simulink model "combinedmodels"  (R2022b)
settings: Solver=VariableStepAuto  StartTime=0.0  StopTime=3600  RelTol=1e-3
libraries: sh_lib x46, spsThreePhaseVIMeasurementLib x36, spsThreePhaseSeriesRLCLoadLib x32, spsThreePhaseSeriesRLCBranchLib x32, fl_lib x27, nesl_utility x25, spsCurrentVoltageSimscapeInterfacegndLib x6, ee_lib x3, spsGroundLib x3, spsPower3phPhasorLib x3, SignalEditorBlockLib x3, spsThreePhaseParallelRLCBranchLib x3
(part 1 of 3)
settings Model: Creator=philip  LastModifiedBy=philip

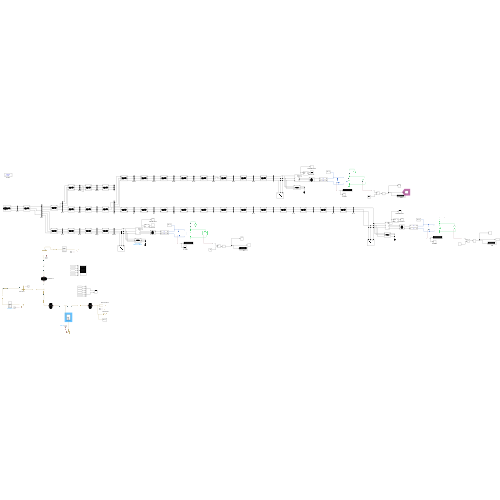
[thumbnail: Simulink's stored preview of the top-level diagram]
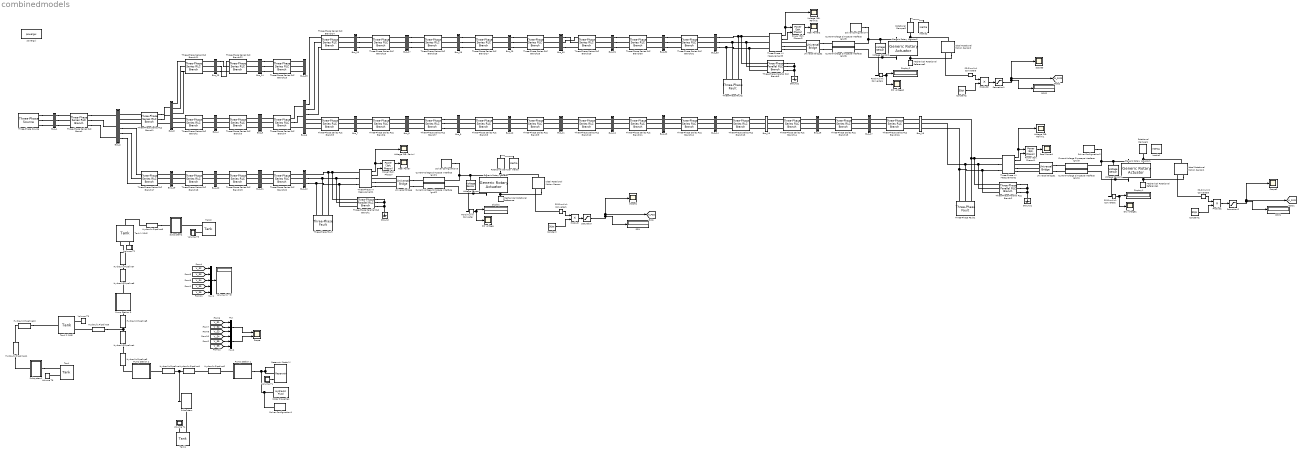
== system combinedmodels ==
  Bus_1 : Subsystem
  Bus_10 : Subsystem
  Bus_11 : Subsystem
  Bus_12 : Subsystem
  Bus_13 : Subsystem
  Bus_14 : Subsystem
  Bus_15 : Subsystem
  Bus_16 : Subsystem
  Bus_17 : Subsystem
  Bus_18 : Subsystem
  Bus_19 : Subsystem
  Bus_2 : Subsystem
  Bus_20 : Subsystem
  Bus_21 : Subsystem
  Bus_22 : Subsystem
  Bus_23 : Subsystem
  Bus_24 : Subsystem
  Bus_25 : Subsystem
  Bus_26 : Subsystem
  Bus_27 : Subsystem
  Bus_28 : Subsystem
  Bus_29 : Subsystem
  Bus_3 : Subsystem
  Bus_30 : Subsystem
  Bus_31 : Subsystem
  Bus_32 : Subsystem
  Bus_33 : Subsystem
  Bus_4 : Subsystem
  Bus_5 : Subsystem
  Bus_6 : Subsystem
  Bus_7 : Subsystem
  Bus_8 : Subsystem
  Bus_9 : Subsystem
  Constant : Constant  Value=30/pi  VectorParams1D=off
  Constant1 : Constant  Value=30/pi  VectorParams1D=off
  Constant2 : Constant  Value=30/pi  VectorParams1D=off
  Current-Voltage Simscape Interface (gnd){1..6} (6 alike) : spsCurrentVoltageSimscapeInterfacegndLib/Current-Voltage Simscape Interface (gnd)  DFT=off  Fmode=Low pass filter (continuous)  T=1e-6  Ts=50e-6  i0=0  v0=12660  Sd=Specialized Power Systems side  Measurements=off
      settings: LibrarySourceBlock=|
      | sps_lib/Utilities/Current-Voltage
      | Simscape Interface
      | (gnd)
  DC voltage : Scope
  DC voltage1 : Scope
  DC voltage2 : Scope
  Display : Display
  Display1 : Display
  Display2 : Display
  Generic Rotary Actuator : ee_lib/Electromechanical/Mechatronic Actuators/Generic Rotary Actuator  w_vec=[-1500, -1000, -500, 0, 500, 1000, 1500, 2000, 2500, 3000] rpm  T_vec=[3.8,3.5, 3, 2.5, 2, 1.5, 1, .5, 0, -.5,] N*m  Vrated=20000 V  eff=60  w_eff=2000 rpm  Pbase=1 W  pwm_or_av=1  J=0.1 kg*m^2  lam=1e-8 N*m/(rad/s)  i_specify=off  i_priority=None  i=0 A  i_nominal_specify=off  i_nominal_unit=A  i_nominal_value=1  t_specify=off  t_priority=None  t=0 N*m  t_nominal_specify=off  t_nominal_unit=N*m  t_nominal_value=1  w_specify=off  w_priority=Low  w=0 rpm  w_nominal_specify=off  w_nominal_unit=rpm  w_nominal_value=1  alpha=3.93e-3 1/K  Tmeas=25 degC  thermal_mass=100 J/K  Q_specify=off  Q_priority=None  Q=0 W  Q_nominal_specify=off  Q_nominal_unit=W  Q_nominal_value=1  temperature_specify=off  temperature_priority=High  temperature=300 K  temperature_nominal_specify=off  temperature_nominal_unit=K  temperature_nominal_value=1
      settings: InternalSimscapePortConfiguration="{\"Bottom\":[],\"Left\":[{\"id\":\"p\",\"label\":\"+\",\"type\":\"foundation.electrical.electrical\"},{\"id\":\"R\",\"label\":\"R\",\"type\":\"foundation.mechanical.rotational.rotational\"}],\"Right\":[{\"id\":\"n\",\"label\":\"-\",\"type\":\"foundation.electrical.electrical\"},{\"id\":\"C\",\"label\":\"C\",\"type\":\"foundation.mechanical.rotational.rotational\"}],\"Top\":[]}"
  Generic Rotary Actuator1 : ee_lib/Electromechanical/Mechatronic Actuators/Generic Rotary Actuator  w_vec=[-1500, -1000, -500, 0, 500, 1000, 1500, 2000, 2500, 3000] rpm  T_vec=[3.8,3.5, 3, 2.5, 2, 1.5, 1, .5, 0, -.5,] N*m  Vrated=20000 V  eff=60  w_eff=2000 rpm  Pbase=1 W  pwm_or_av=1  J=0.1 kg*m^2  lam=1e-8 N*m/(rad/s)  i_specify=off  i_priority=None  i=0 A  i_nominal_specify=off  i_nominal_unit=A  i_nominal_value=1  t_specify=off  t_priority=None  t=0 N*m  t_nominal_specify=off  t_nominal_unit=N*m  t_nominal_value=1  w_specify=off  w_priority=Low  w=0 rpm  w_nominal_specify=off  w_nominal_unit=rpm  w_nominal_value=1  alpha=3.93e-3 1/K  Tmeas=25 degC  thermal_mass=100 J/K  Q_specify=off  Q_priority=None  Q=0 W  Q_nominal_specify=off  Q_nominal_unit=W  Q_nominal_value=1  temperature_specify=off  temperature_priority=High  temperature=300 K  temperature_nominal_specify=off  temperature_nominal_unit=K  temperature_nominal_value=1
      settings: InternalSimscapePortConfiguration="{\"Bottom\":[],\"Left\":[{\"id\":\"p\",\"label\":\"+\",\"type\":\"foundation.electrical.electrical\"},{\"id\":\"R\",\"label\":\"R\",\"type\":\"foundation.mechanical.rotational.rotational\"}],\"Right\":[{\"id\":\"n\",\"label\":\"-\",\"type\":\"foundation.electrical.electrical\"},{\"id\":\"C\",\"label\":\"C\",\"type\":\"foundation.mechanical.rotational.rotational\"}],\"Top\":[]}"
  Generic Rotary Actuator2 : ee_lib/Electromechanical/Mechatronic Actuators/Generic Rotary Actuator  w_vec=[-1500, -1000, -500, 0, 500, 1000, 1500, 2000, 2500, 3000] rpm  T_vec=[3.8,3.5, 3, 2.5, 2, 1.5, 1, .5, 0, -.5,] N*m  Vrated=20000 V  eff=60  w_eff=2000 rpm  Pbase=1 W  pwm_or_av=1  J=0.1 kg*m^2  lam=1e-8 N*m/(rad/s)  i_specify=off  i_priority=None  i=0 A  i_nominal_specify=off  i_nominal_unit=A  i_nominal_value=1  t_specify=off  t_priority=None  t=0 N*m  t_nominal_specify=off  t_nominal_unit=N*m  t_nominal_value=1  w_specify=off  w_priority=Low  w=0 rpm  w_nominal_specify=off  w_nominal_unit=rpm  w_nominal_value=1  alpha=3.93e-3 1/K  Tmeas=25 degC  thermal_mass=100 J/K  Q_specify=off  Q_priority=None  Q=0 W  Q_nominal_specify=off  Q_nominal_unit=W  Q_nominal_value=1  temperature_specify=off  temperature_priority=High  temperature=300 K  temperature_nominal_specify=off  temperature_nominal_unit=K  temperature_nominal_value=1
      settings: InternalSimscapePortConfiguration="{\"Bottom\":[],\"Left\":[{\"id\":\"p\",\"label\":\"+\",\"type\":\"foundation.electrical.electrical\"},{\"id\":\"R\",\"label\":\"R\",\"type\":\"foundation.mechanical.rotational.rotational\"}],\"Right\":[{\"id\":\"n\",\"label\":\"-\",\"type\":\"foundation.electrical.electrical\"},{\"id\":\"C\",\"label\":\"C\",\"type\":\"foundation.mechanical.rotational.rotational\"}],\"Top\":[]}"
  Ground : spsGroundLib/Ground  LConnTagsString=a
  Ground1 : spsGroundLib/Ground  LConnTagsString=a
  Ground2 : spsGroundLib/Ground  LConnTagsString=a
  Hydraulic Pipeline : sh_lib/Pipelines/Hydraulic Pipeline  cs_type=foundation.enum.pipeCrossSection.circular  d_in=0.30 m  area=1e-4 m^2  D_h=1.12e-2 m  s_factor=64  length=18 m  length_ad=1 m  roughness=15e-6 m  Re_lam=2000  Re_turb=4000  wall_type=foundation.enum.chamber_spec.rigid  pr_r_coef=2e-12 m/Pa  time_const=0.01 s  k_sh=1.4  initial_pressure=0 Pa
      settings: InternalSimscapePortConfiguration="{\"Bottom\":[],\"Left\":[{\"id\":\"A\",\"label\":\"A\",\"type\":\"foundation.hydraulic.hydraulic\"}],\"Right\":[{\"id\":\"B\",\"label\":\"B\",\"type\":\"foundation.hydraulic.hydraulic\"}],\"Top\":[]}"
  Hydraulic Pipeline1 : sh_lib/Pipelines/Hydraulic Pipeline  cs_type=foundation.enum.pipeCrossSection.circular  d_in=0.15 m  area=1e-4 m^2  D_h=1.12e-2 m  s_factor=64  length=401 m  length_ad=1 m  roughness=15e-6 m  Re_lam=2000  Re_turb=4000  wall_type=foundation.enum.chamber_spec.rigid  pr_r_coef=2e-12 m/Pa  time_const=0.01 s  k_sh=1.4  initial_pressure=0 Pa
      settings: InternalSimscapePortConfiguration="{\"Bottom\":[],\"Left\":[{\"id\":\"A\",\"label\":\"A\",\"type\":\"foundation.hydraulic.hydraulic\"}],\"Right\":[{\"id\":\"B\",\"label\":\"B\",\"type\":\"foundation.hydraulic.hydraulic\"}],\"Top\":[]}"
  Hydraulic Pipeline10 : sh_lib/Pipelines/Hydraulic Pipeline  cs_type=foundation.enum.pipeCrossSection.circular  d_in=0.23 m  area=1e-4 m^2  D_h=1.12e-2 m  s_factor=64  length=6 m  length_ad=1 m  roughness=15e-6 m  Re_lam=2000  Re_turb=4000  wall_type=foundation.enum.chamber_spec.rigid  pr_r_coef=2e-12 m/Pa  time_const=0.01 s  k_sh=1.4  initial_pressure=0 Pa
      settings: InternalSimscapePortConfiguration="{\"Bottom\":[],\"Left\":[{\"id\":\"A\",\"label\":\"A\",\"type\":\"foundation.hydraulic.hydraulic\"}],\"Right\":[{\"id\":\"B\",\"label\":\"B\",\"type\":\"foundation.hydraulic.hydraulic\"}],\"Top\":[]}"
  Hydraulic Pipeline11 : sh_lib/Pipelines/Hydraulic Pipeline  cs_type=foundation.enum.pipeCrossSection.circular  d_in=0.30 m  area=1e-4 m^2  D_h=1.12e-2 m  s_factor=64  length=13 m  length_ad=1 m  roughness=15e-6 m  Re_lam=2000  Re_turb=4000  wall_type=foundation.enum.chamber_spec.rigid  pr_r_coef=2e-12 m/Pa  time_const=0.01 s  k_sh=1.4  initial_pressure=0 Pa
      settings: InternalSimscapePortConfiguration="{\"Bottom\":[],\"Left\":[{\"id\":\"A\",\"label\":\"A\",\"type\":\"foundation.hydraulic.hydraulic\"}],\"Right\":[{\"id\":\"B\",\"label\":\"B\",\"type\":\"foundation.hydraulic.hydraulic\"}],\"Top\":[]}"
  Hydraulic Pipeline2 : sh_lib/Pipelines/Hydraulic Pipeline  cs_type=foundation.enum.pipeCrossSection.circular  d_in=0.15 m  area=1e-4 m^2  D_h=1.12e-2 m  s_factor=64  length=15 m  length_ad=1 m  roughness=15e-6 m  Re_lam=2000  Re_turb=4000  wall_type=foundation.enum.chamber_spec.rigid  pr_r_coef=2e-12 m/Pa  time_const=0.01 s  k_sh=1.4  initial_pressure=0 Pa
      settings: InternalSimscapePortConfiguration="{\"Bottom\":[],\"Left\":[{\"id\":\"A\",\"label\":\"A\",\"type\":\"foundation.hydraulic.hydraulic\"}],\"Right\":[{\"id\":\"B\",\"label\":\"B\",\"type\":\"foundation.hydraulic.hydraulic\"}],\"Top\":[]}"
  Hydraulic Pipeline3 : sh_lib/Pipelines/Hydraulic Pipeline  cs_type=foundation.enum.pipeCrossSection.circular  d_in=0.25 m  area=1e-4 m^2  D_h=1.12e-2 m  s_factor=64  length=1087 m  length_ad=1 m  roughness=15e-6 m  Re_lam=2000  Re_turb=4000  wall_type=foundation.enum.chamber_spec.rigid  pr_r_coef=2e-12 m/Pa  time_const=0.01 s  k_sh=1.4  initial_pressure=0 Pa
      settings: InternalSimscapePortConfiguration="{\"Bottom\":[],\"Left\":[{\"id\":\"A\",\"label\":\"A\",\"type\":\"foundation.hydraulic.hydraulic\"}],\"Right\":[{\"id\":\"B\",\"label\":\"B\",\"type\":\"foundation.hydraulic.hydraulic\"}],\"Top\":[]}"
  Hydraulic Pipeline4 : sh_lib/Pipelines/Hydraulic Pipeline  cs_type=foundation.enum.pipeCrossSection.circular  d_in=0.15 m  area=1e-4 m^2  D_h=1.12e-2 m  s_factor=64  length=1002 m  length_ad=1 m  roughness=15e-6 m  Re_lam=2000  Re_turb=4000  wall_type=foundation.enum.chamber_spec.rigid  pr_r_coef=2e-12 m/Pa  time_const=0.01 s  k_sh=1.4  initial_pressure=0 Pa
      settings: InternalSimscapePortConfiguration="{\"Bottom\":[],\"Left\":[{\"id\":\"A\",\"label\":\"A\",\"type\":\"foundation.hydraulic.hydraulic\"}],\"Right\":[{\"id\":\"B\",\"label\":\"B\",\"type\":\"foundation.hydraulic.hydraulic\"}],\"Top\":[]}"
  Hydraulic Pipeline5 : sh_lib/Pipelines/Hydraulic Pipeline  cs_type=foundation.enum.pipeCrossSection.circular  d_in=0.10 m  area=1e-4 m^2  D_h=1.12e-2 m  s_factor=64  length=846 m  length_ad=1 m  roughness=15e-6 m  Re_lam=2000  Re_turb=4000  wall_type=foundation.enum.chamber_spec.rigid  pr_r_coef=2e-12 m/Pa  time_const=0.01 s  k_sh=1.4  initial_pressure=0 Pa
      settings: InternalSimscapePortConfiguration="{\"Bottom\":[],\"Left\":[{\"id\":\"A\",\"label\":\"A\",\"type\":\"foundation.hydraulic.hydraulic\"}],\"Right\":[{\"id\":\"B\",\"label\":\"B\",\"type\":\"foundation.hydraulic.hydraulic\"}],\"Top\":[]}"
  Hydraulic Pipeline6 : sh_lib/Pipelines/Hydraulic Pipeline  cs_type=foundation.enum.pipeCrossSection.circular  d_in=0.25 m  area=1e-4 m^2  D_h=1.12e-2 m  s_factor=64  length=44 m  length_ad=1 m  roughness=15e-6 m  Re_lam=2000  Re_turb=4000  wall_type=foundation.enum.chamber_spec.rigid  pr_r_coef=2e-12 m/Pa  time_const=0.01 s  k_sh=1.4  initial_pressure=0 Pa
      settings: InternalSimscapePortConfiguration="{\"Bottom\":[],\"Left\":[{\"id\":\"A\",\"label\":\"A\",\"type\":\"foundation.hydraulic.hydraulic\"}],\"Right\":[{\"id\":\"B\",\"label\":\"B\",\"type\":\"foundation.hydraulic.hydraulic\"}],\"Top\":[]}"
  Hydraulic Pipeline7 : sh_lib/Pipelines/Hydraulic Pipeline  cs_type=foundation.enum.pipeCrossSection.circular  d_in=0.25 m  area=1e-4 m^2  D_h=1.12e-2 m  s_factor=64  length=18 m  length_ad=1 m  roughness=15e-6 m  Re_lam=2000  Re_turb=4000  wall_type=foundation.enum.chamber_spec.rigid  pr_r_coef=2e-12 m/Pa  time_const=0.01 s  k_sh=1.4  initial_pressure=0 Pa
      settings: InternalSimscapePortConfiguration="{\"Bottom\":[],\"Left\":[{\"id\":\"A\",\"label\":\"A\",\"type\":\"foundation.hydraulic.hydraulic\"}],\"Right\":[{\"id\":\"B\",\"label\":\"B\",\"type\":\"foundation.hydraulic.hydraulic\"}],\"Top\":[]}"
  Hydraulic Pipeline8 : sh_lib/Pipelines/Hydraulic Pipeline  cs_type=foundation.enum.pipeCrossSection.circular  d_in=0.10 m  area=1e-4 m^2  D_h=1.12e-2 m  s_factor=64  length=16 m  length_ad=1 m  roughness=15e-6 m  Re_lam=2000  Re_turb=4000  wall_type=foundation.enum.chamber_spec.rigid  pr_r_coef=2e-12 m/Pa  time_const=0.01 s  k_sh=1.4  initial_pressure=0 Pa
      settings: InternalSimscapePortConfiguration="{\"Bottom\":[],\"Left\":[{\"id\":\"A\",\"label\":\"A\",\"type\":\"foundation.hydraulic.hydraulic\"}],\"Right\":[{\"id\":\"B\",\"label\":\"B\",\"type\":\"foundation.hydraulic.hydraulic\"}],\"Top\":[]}"
  Hydraulic Pipeline9 : sh_lib/Pipelines/Hydraulic Pipeline  cs_type=foundation.enum.pipeCrossSection.circular  d_in=0.20 m  area=1e-4 m^2  D_h=1.12e-2 m  s_factor=64  length=1003 m  length_ad=1 m  roughness=15e-6 m  Re_lam=2000  Re_turb=4000  wall_type=foundation.enum.chamber_spec.rigid  pr_r_coef=2e-12 m/Pa  time_const=0.01 s  k_sh=1.4  initial_pressure=0 Pa
      settings: InternalSimscapePortConfiguration="{\"Bottom\":[],\"Left\":[{\"id\":\"A\",\"label\":\"A\",\"type\":\"foundation.hydraulic.hydraulic\"}],\"Right\":[{\"id\":\"B\",\"label\":\"B\",\"type\":\"foundation.hydraulic.hydraulic\"}],\"Top\":[]}"
  Ideal Rotational Motion Sensor : fl_lib/Mechanical/Mechanical Sensors/Ideal Rotational Motion Sensor  reference=foundation.enum.MeasurementReference.difference  acceleration_port=false  velocity_port=true  position_port=false  wrap_angle=false  offset=0 rad
      settings: InternalSimscapePortConfiguration="{\"Bottom\":[],\"Left\":[{\"id\":\"R\",\"label\":\"R\",\"type\":\"foundation.mechanical.rotational.rotational\"}],\"Right\":[{\"id\":\"C\",\"label\":\"C\",\"type\":\"foundation.mechanical.rotational.rotational\"},{\"id\":\"W\",\"label\":\"W\",\"type\":\"output\"}],\"Top\":[]}"
  Ideal Rotational Motion Sensor1 : fl_lib/Mechanical/Mechanical Sensors/Ideal Rotational Motion Sensor  reference=foundation.enum.MeasurementReference.difference  acceleration_port=false  velocity_port=true  position_port=false  wrap_angle=false  offset=0 rad
      settings: InternalSimscapePortConfiguration="{\"Bottom\":[],\"Left\":[{\"id\":\"R\",\"label\":\"R\",\"type\":\"foundation.mechanical.rotational.rotational\"}],\"Right\":[{\"id\":\"C\",\"label\":\"C\",\"type\":\"foundation.mechanical.rotational.rotational\"},{\"id\":\"W\",\"label\":\"W\",\"type\":\"output\"}],\"Top\":[]}"
  Ideal Rotational Motion Sensor2 : fl_lib/Mechanical/Mechanical Sensors/Ideal Rotational Motion Sensor  reference=foundation.enum.MeasurementReference.difference  acceleration_port=false  velocity_port=true  position_port=false  wrap_angle=false  offset=0 rad
      settings: InternalSimscapePortConfiguration="{\"Bottom\":[],\"Left\":[{\"id\":\"R\",\"label\":\"R\",\"type\":\"foundation.mechanical.rotational.rotational\"}],\"Right\":[{\"id\":\"C\",\"label\":\"C\",\"type\":\"foundation.mechanical.rotational.rotational\"},{\"id\":\"W\",\"label\":\"W\",\"type\":\"output\"}],\"Top\":[]}"
  Inertia : fl_lib/Mechanical/Rotational Elements/Inertia  inertia=0.1 kg*m^2  num_ports=foundation.enum.numPorts2.one  w_specify=off  w_priority=High  w=0 rad/s  w_nominal_specify=off  w_nominal_unit=rad/s  w_nominal_value=1  t_specify=off  t_priority=None  t=0 N*m  t_nominal_specify=off  t_nominal_unit=N*m  t_nominal_value=1
  Inertia1 : fl_lib/Mechanical/Rotational Elements/Inertia  inertia=0.1 kg*m^2  num_ports=foundation.enum.numPorts2.one  w_specify=off  w_priority=High  w=0 rad/s  w_nominal_specify=off  w_nominal_unit=rad/s  w_nominal_value=1  t_specify=off  t_priority=None  t=0 N*m  t_nominal_specify=off  t_nominal_unit=N*m  t_nominal_value=1
  Inertia2 : fl_lib/Mechanical/Rotational Elements/Inertia  inertia=0.1 kg*m^2  num_ports=foundation.enum.numPorts2.one  w_specify=off  w_priority=High  w=0 rad/s  w_nominal_specify=off  w_nominal_unit=rad/s  w_nominal_value=1  t_specify=off  t_priority=None  t=0 N*m  t_nominal_specify=off  t_nominal_unit=N*m  t_nominal_value=1
  Mechanical Rotational Reference : fl_lib/Mechanical/Rotational Elements/Mechanical Rotational Reference
  Mechanical Rotational Reference1 : fl_lib/Mechanical/Rotational Elements/Mechanical Rotational Reference
  Mechanical Rotational Reference2 : fl_lib/Mechanical/Rotational Elements/Mechanical Rotational Reference
  Mux : Mux  Inputs=3
  Mux1 : Mux  Inputs=5
  Mux2 : Mux  Inputs=3
  PS-Simulink Converter : nesl_utility/PS-Simulink Converter  PhysicalDomain=network_engine_domain  SubClassName=ps_output  LeftPortType=input  RightPortType=output  PseudoPeriodic=off  Frequencies=[]  VectorFormat=1-D array  Unit=inherit  AffineConversion=off
  PS-Simulink Converter1 : nesl_utility/PS-Simulink Converter  PhysicalDomain=network_engine_domain  SubClassName=ps_output  LeftPortType=input  RightPortType=output  PseudoPeriodic=off  Frequencies=[]  VectorFormat=inherit  Unit=inherit  AffineConversion=off
  PS-Simulink Converter2 : nesl_utility/PS-Simulink Converter  PhysicalDomain=network_engine_domain  SubClassName=ps_output  LeftPortType=input  RightPortType=output  PseudoPeriodic=off  Frequencies=[]  VectorFormat=1-D array  Unit=inherit  AffineConversion=off
  PS-Simulink Converter3 : nesl_utility/PS-Simulink Converter  PhysicalDomain=network_engine_domain  SubClassName=ps_output  LeftPortType=input  RightPortType=output  PseudoPeriodic=off  Frequencies=[]  VectorFormat=inherit  Unit=inherit  AffineConversion=off
  PS-Simulink Converter4 : nesl_utility/PS-Simulink Converter  PhysicalDomain=network_engine_domain  SubClassName=ps_output  LeftPortType=input  RightPortType=output  PseudoPeriodic=off  Frequencies=[]  VectorFormat=1-D array  Unit=inherit  AffineConversion=off
  PS-Simulink Converter5 : nesl_utility/PS-Simulink Converter  PhysicalDomain=network_engine_domain  SubClassName=ps_output  LeftPortType=input  RightPortType=output  PseudoPeriodic=off  Frequencies=[]  VectorFormat=inherit  Unit=inherit  AffineConversion=off
  "Power (3ph, Phasor)" : spsPower3phPhasorLib/Power (3ph, Phasor)
      settings: LibrarySourceBlock=|
      | sps_lib/Sensors and Measurements/Power
      | (3ph, Phasor)
  "Power (3ph, Phasor)1" : spsPower3phPhasorLib/Power (3ph, Phasor)
      settings: LibrarySourceBlock=|
      | sps_lib/Sensors and Measurements/Power
      | (3ph, Phasor)
  "Power (3ph, Phasor)2" : spsPower3phPhasorLib/Power (3ph, Phasor)
      settings: LibrarySourceBlock=|
      | sps_lib/Sensors and Measurements/Power
      | (3ph, Phasor)
  Product : Product
  Product1 : Product
  Product2 : Product
  Pump Station 1 : Subsystem  Tag=PublishSubsystem
      mask Display:
      | plot(sin(0:0.5:4.5*pi)*0.9, cos(0:0.5:4.5*pi)*0.9+1.5)
      | plot(sin(0:0.5:4.5*pi)*0.5, cos(0:0.5:4.5*pi)*0.5+1.5)
      | plot(sin(0:0.5:4.5*pi)*0.9, cos(0:0.5:4.5*pi)*0.9-1.5)
      | plot(sin(0:0.5:4.5*pi)*0.5, cos(0:0.5:4.5*pi)*0.5-1.5)
      | 
      | plot([0 -0.9],[1.5 1.5-0.9])
      | plot([0 -0.9],[1.5 1.5-0.9]*-1)
      | 
      | plot([0.45 0.45 0.325 0.325]*2,[1.5 1.5-1.0 1.5-1.0 1.5-0.55])
      | plot([0.45 0.45 0.325 0.325]*2,[1.5 1.5-0.9 1.5-0.9 1.5-0.55]*-1)
      | 
      | plot([2.2 0.95]*-1,[0 0])
      | plot([2.2 0.95],[0 0])
      | 
      | plot([0.95 0.95]*-1,[-0.6 0.6])
      | plot([0.8 0.8],[-0.55 0.55])
      | 
      | 
      | color('white');plot(-3,-2.5);plot(3,2.5);
      | color('red');
      | port_label('LConn',1,'T');
      | port_label('RConn',1,'P');
  Pump Station 2 : Subsystem  Tag=PublishSubsystem
      mask Display:
      | plot(sin(0:0.5:4.5*pi)*0.9, cos(0:0.5:4.5*pi)*0.9+1.5)
      | plot(sin(0:0.5:4.5*pi)*0.5, cos(0:0.5:4.5*pi)*0.5+1.5)
      | plot(sin(0:0.5:4.5*pi)*0.9, cos(0:0.5:4.5*pi)*0.9-1.5)
      | plot(sin(0:0.5:4.5*pi)*0.5, cos(0:0.5:4.5*pi)*0.5-1.5)
      | 
      | plot([0 -0.9],[1.5 1.5-0.9])
      | plot([0 -0.9],[1.5 1.5-0.9]*-1)
      | 
      | plot([0.45 0.45 0.325 0.325]*2,[1.5 1.5-1.0 1.5-1.0 1.5-0.55])
      | plot([0.45 0.45 0.325 0.325]*2,[1.5 1.5-0.9 1.5-0.9 1.5-0.55]*-1)
      | 
      | plot([2.2 0.95]*-1,[0 0])
      | plot([2.2 0.95],[0 0])
      | 
      | plot([0.95 0.95]*-1,[-0.6 0.6])
      | plot([0.8 0.8],[-0.55 0.55])
      | 
      | 
      | color('white');plot(-3,-2.5);plot(3,2.5);
      | color('red');
      | port_label('LConn',1,'T');
      | port_label('RConn',1,'P');
  Pump Station 3 : Subsystem  Tag=PublishSubsystem
      mask Display:
      | plot(sin(0:0.5:4.5*pi)*0.9, cos(0:0.5:4.5*pi)*0.9+1.5)
      | plot(sin(0:0.5:4.5*pi)*0.5, cos(0:0.5:4.5*pi)*0.5+1.5)
      | plot(sin(0:0.5:4.5*pi)*0.9, cos(0:0.5:4.5*pi)*0.9-1.5)
      | plot(sin(0:0.5:4.5*pi)*0.5, cos(0:0.5:4.5*pi)*0.5-1.5)
      | 
      | plot([0 -0.9],[1.5 1.5-0.9])
      | plot([0 -0.9],[1.5 1.5-0.9]*-1)
      | 
      | plot([0.45 0.45 0.325 0.325]*2,[1.5 1.5-1.0 1.5-1.0 1.5-0.55])
      | plot([0.45 0.45 0.325 0.325]*2,[1.5 1.5-0.9 1.5-0.9 1.5-0.55]*-1)
      | 
      | plot([2.2 0.95]*-1,[0 0])
      | plot([2.2 0.95],[0 0])
      | 
      | plot([0.95 0.95]*-1,[-0.6 0.6])
      | plot([0.8 0.8],[-0.55 0.55])
      | 
      | 
      | color('white');plot(-3,-2.5);plot(3,2.5);
      | color('red');
      | port_label('LConn',1,'T');
      | port_label('RConn',1,'P');
  RPM : Display
  RPM1 : Display
  RPM2 : Display
  Real Power : Scope
  Real Power1 : Scope
  Real Power2 : Scope
  Reservoir (Node 1) : sh_lib/Hydraulic Utilities/Reservoir  press=0 Pa  init_volume=200 m^3  ret_diam=0.15 m  loss_coeff=1
      settings: InternalSimscapePortConfiguration="{\"Bottom\":[],\"Left\":[{\"id\":\"V\",\"label\":\"V\",\"type\":\"output\"},{\"id\":\"P\",\"label\":\"P\",\"type\":\"foundation.hydraulic.hydraulic\"},{\"id\":\"R\",\"label\":\"R\",\"type\":\"foundation.hydraulic.hydraulic\"}],\"Right\":[],\"Top\":[]}"
  Rotational Damper : fl_lib/Mechanical/Rotational Elements/Rotational Damper  D=0.001 N*m/(rad/s)  w_specify=off  w_priority=None  w=0 rad/s  w_nominal_specify=off  w_nominal_unit=rad/s  w_nominal_value=1  t_specify=off  t_priority=None  t=0 N*m  t_nominal_specify=off  t_nominal_unit=N*m  t_nominal_value=1
  Rotational Damper1 : fl_lib/Mechanical/Rotational Elements/Rotational Damper  D=0.001 N*m/(rad/s)  w_specify=off  w_priority=None  w=0 rad/s  w_nominal_specify=off  w_nominal_unit=rad/s  w_nominal_value=1  t_specify=off  t_priority=None  t=0 N*m  t_nominal_specify=off  t_nominal_unit=N*m  t_nominal_value=1
  Rotational Damper2 : fl_lib/Mechanical/Rotational Elements/Rotational Damper  D=0.001 N*m/(rad/s)  w_specify=off  w_priority=None  w=0 rad/s  w_nominal_specify=off  w_nominal_unit=rad/s  w_nominal_value=1  t_specify=off  t_priority=None  t=0 N*m  t_nominal_specify=off  t_nominal_unit=N*m  t_nominal_value=1
  Saturation : Saturate  UpperLimit=2500  LowerLimit=0  OutMin=[0]  OutMax=[2500]
  Saturation1 : Saturate  UpperLimit=2500  LowerLimit=0  OutMin=[0]  OutMax=[2500]
  Saturation2 : Saturate  UpperLimit=2500  LowerLimit=0  OutMin=[0]  OutMax=[2500]
  Scope : Scope  NumInputPorts=2
  Scope1 : Scope
  Scope2 : Scope
  Scope3 : Scope
  Solver Configuration1 : nesl_utility/Solver Configuration  PhysicalDomain=network_engine_domain  SubClassName=solver  LeftPortType=input  RightPortType=generic  Tones=[]  Harmonics=[]  SimulateNoise=off  Profile=off  UseLocalSampling=off  EnableSwitchedLinearOptims=on  FrequencyDomain=off  UseCCode=off  RelTol=0.001  AbsTol=1e-06  MinStep=1e-09  ToWorkspace=off  RevertToSquareIcSolve=off  NumHomotopyIterations=100  PhasorMode=off  PhasorModeNumHarmonics=1  ConsistencySolver=NEWTON_XTOL_AFTER_FTOL  IndexReductionMethod=DerivativeReplacement  DoDC=off  ResidualTolerance=1e-9  ConsistencyTolSource=GLOBAL  ConsistencyAbsTol=0.001  ConsistencyRelTol=0.001  ConsistencyTolFactor=0.034  UseLocalSolver=off  LocalSolverChoice=NE_BACKWARD_EULER_ADVANCER  ResolveIndetEquations=on  FunctionEvalNumThread=1  LocalSolverSampleTime=.001  DoFixedCost=on  MaxNonlinIter=3  MaxModeIter=2  ComputeImpulses=off  ImpulseIterations=2  LinearAlgebra=auto  LinearAlgebraNumThread=0  EquationFormulation=NE_TIME_EF  DelaysMemoryBudget=1024  AutomaticFiltering=off  FilteringTimeConstant=0.0001  PartitionStorageMethod=AS_NEEDED  PartitionMemoryBudget=1024  PartitionMethod=FAST
  Solver Configuration2 : nesl_utility/Solver Configuration  PhysicalDomain=network_engine_domain  SubClassName=solver  LeftPortType=input  RightPortType=generic  Tones=[]  Harmonics=[]  SimulateNoise=off  Profile=off  UseLocalSampling=off  EnableSwitchedLinearOptims=on  FrequencyDomain=off  UseCCode=off  RelTol=0.001  AbsTol=1e-06  MinStep=1e-09  ToWorkspace=off  RevertToSquareIcSolve=off  NumHomotopyIterations=100  PhasorMode=off  PhasorModeNumHarmonics=1  ConsistencySolver=NEWTON_FTOL  IndexReductionMethod=DerivativeReplacement  DoDC=off  ResidualTolerance=1e-09  ConsistencyTolSource=GLOBAL  ConsistencyAbsTol=0.001  ConsistencyRelTol=0.001  ConsistencyTolFactor=0.001  UseLocalSolver=off  LocalSolverChoice=NE_BACKWARD_EULER_ADVANCER  ResolveIndetEquations=on  FunctionEvalNumThread=1  LocalSolverSampleTime=0.001  DoFixedCost=off  MaxNonlinIter=3  MaxModeIter=2  ComputeImpulses=off  ImpulseIterations=2  LinearAlgebra=auto  LinearAlgebraNumThread=0  EquationFormulation=NE_TIME_EF  DelaysMemoryBudget=1024  AutomaticFiltering=on  FilteringTimeConstant=0.001  PartitionStorageMethod=AS_NEEDED  PartitionMemoryBudget=1024  PartitionMethod=ROBUST
  Solver Configuration3 : nesl_utility/Solver Configuration  PhysicalDomain=network_engine_domain  SubClassName=solver  LeftPortType=input  RightPortType=generic  Tones=[]  Harmonics=[]  SimulateNoise=off  Profile=off  UseLocalSampling=off  EnableSwitchedLinearOptims=on  FrequencyDomain=off  UseCCode=off  RelTol=0.001  AbsTol=1e-06  MinStep=1e-09  ToWorkspace=off  RevertToSquareIcSolve=off  NumHomotopyIterations=100  PhasorMode=off  PhasorModeNumHarmonics=1  ConsistencySolver=NEWTON_FTOL  IndexReductionMethod=DerivativeReplacement  DoDC=off  ResidualTolerance=1e-09  ConsistencyTolSource=GLOBAL  ConsistencyAbsTol=0.001  ConsistencyRelTol=0.001  ConsistencyTolFactor=0.001  UseLocalSolver=off  LocalSolverChoice=NE_BACKWARD_EULER_ADVANCER  ResolveIndetEquations=on  FunctionEvalNumThread=1  LocalSolverSampleTime=0.001  DoFixedCost=off  MaxNonlinIter=3  MaxModeIter=2  ComputeImpulses=off  ImpulseIterations=2  LinearAlgebra=auto  LinearAlgebraNumThread=0  EquationFormulation=NE_TIME_EF  DelaysMemoryBudget=1024  AutomaticFiltering=on  FilteringTimeConstant=0.001  PartitionStorageMethod=AS_NEEDED  PartitionMemoryBudget=1024  PartitionMethod=ROBUST
  Solver Configuration4 : nesl_utility/Solver Configuration  PhysicalDomain=network_engine_domain  SubClassName=solver  LeftPortType=input  RightPortType=generic  Tones=[]  Harmonics=[]  SimulateNoise=off  Profile=off  UseLocalSampling=off  EnableSwitchedLinearOptims=on  FrequencyDomain=off  UseCCode=off  RelTol=0.001  AbsTol=1e-06  MinStep=1e-09  ToWorkspace=off  RevertToSquareIcSolve=off  NumHomotopyIterations=100  PhasorMode=off  PhasorModeNumHarmonics=1  ConsistencySolver=NEWTON_FTOL  IndexReductionMethod=DerivativeReplacement  DoDC=off  ResidualTolerance=1e-09  ConsistencyTolSource=GLOBAL  ConsistencyAbsTol=0.001  ConsistencyRelTol=0.001  ConsistencyTolFactor=0.001  UseLocalSolver=off  LocalSolverChoice=NE_BACKWARD_EULER_ADVANCER  ResolveIndetEquations=on  FunctionEvalNumThread=1  LocalSolverSampleTime=0.001  DoFixedCost=off  MaxNonlinIter=3  MaxModeIter=2  ComputeImpulses=off  ImpulseIterations=2  LinearAlgebra=auto  LinearAlgebraNumThread=0  EquationFormulation=NE_TIME_EF  DelaysMemoryBudget=1024  AutomaticFiltering=on  FilteringTimeConstant=0.001  PartitionStorageMethod=AS_NEEDED  PartitionMemoryBudget=1024  PartitionMethod=ROBUST
  Subsystem : Subsystem
      settings: PortSchema="{\"entries\":[{\"content\":{\"sides\":[{\"content\":{\"connectorIds\":[\"LConn1\"]},\"type\":\"ConnectorPlacement.EquallySpacedRectSide\",\"uuid\":\"c5da6f35-8fa4-48b7-8a4a-4ae9db04ca9d\"},{\"content\":{\"connectorIds\":[],\"side\":\"RIGHT\"},\"type\":\"ConnectorPlacement.EquallySpacedRectSide\",\"uuid\":\"484dc1ab-2dc7-464f-80da-36af203a6e69\"},{\"content\":{\"connectorIds\":[],\"side\":\"TOP\"},\"type\":\"ConnectorPlacement.EquallySpacedRectSide\",\"uuid\":\"15bf6548-86e0-4373-a220-3fe0e1067d73\"},{\"content\":{\"connectorIds\":[\"RConn1\"],\"side\":\"BOTTOM\"},\"type\":\"ConnectorPlacement.EquallySpacedRectSide\",\"uuid\":\"b94051b1-e6bf-4793-98e6-5d6956093d36\"}]},\"type\":\"ConnectorPlacement.EquallySpacedConnector\",\"uuid\":\"b1159124-f196-4e4e-b402-5d78480e647c\"}],\"packageUris\":[\"http://schema.mathworks.com/mf0/Connector/R2020b\"],\"version\":\"1.0\"}"
  Subsystem1 : Subsystem
  Subsystem2 : Subsystem
  Tank : sh_lib/Low-Pressure Blocks/Tank  press=0 Pa  level_spec=1  tank_area=0.8 m^2  fluid_volume_tab=[0, .0028, .0065, .0114, .0176, .0252, .0344, .0436, .0512, .0574, .0623, .066, .0688, .0707, .072, .0727] m^3  fluid_level_tab=[0, .02, .04, .06, .08, .1, .12, .14, .16, .18, .2, .22, .24, .26, .28, .3] m  interp_method=1  extrap_method=1  pipe_diam=0.10 m  loss_coeff=1.2  g=9.80665 m/s^2  min_level=1e-3 m  fluid_level_check=0  volume_specify=off  volume_priority=High  volume=20 l  volume_nominal_specify=off  volume_nominal_unit=l  volume_nominal_value=1  level_specify=off  level_priority=None  level=0.025 m  level_nominal_specify=off  level_nominal_unit=m  level_nominal_value=1  pipe_diam_A=0.02 m  loss_coeff_A=1.2  height_B=0.8 m  pipe_diam_B=0.02 m  loss_coeff_B=1.2  height_C=0.8 m  pipe_diam_C=0.02 m  loss_coeff_C=1.2
      settings: InternalSimscapePortConfiguration="{\"Bottom\":[],\"Left\":[],\"Right\":[{\"id\":\"V\",\"label\":\"V\",\"type\":\"output\"},{\"id\":\"T\",\"label\":\"T\",\"type\":\"foundation.hydraulic.hydraulic\"}],\"Top\":[]}"
  Tank 1 (N10) : sh_lib/Low-Pressure Blocks/Tank  press=0 Pa  level_spec=1  tank_area=0.8 m^2  fluid_volume_tab=[0, .0028, .0065, .0114, .0176, .0252, .0344, .0436, .0512, .0574, .0623, .066, .0688, .0707, .072, .0727] m^3  fluid_level_tab=[0, .02, .04, .06, .08, .1, .12, .14, .16, .18, .2, .22, .24, .26, .28, .3] m  interp_method=1  extrap_method=1  pipe_diam=0.02 m  loss_coeff=1.2  g=9.80665 m/s^2  min_level=1e-3 m  fluid_level_check=0  volume_specify=off  volume_priority=High  volume=100 m^3  volume_nominal_specify=off  volume_nominal_unit=l  volume_nominal_value=1  level_specify=off  level_priority=None  level=station_3.fluid_level m  level_nominal_specify=off  level_nominal_unit=m  level_nominal_value=1  pipe_diam_A=0.25 m  loss_coeff_A=1.2  height_B=0.8 m  pipe_diam_B=0.10 m  loss_coeff_B=1.2  height_C=0.8 m  pipe_diam_C=0.02 m  loss_coeff_C=1.2
      settings: InternalSimscapePortConfiguration="{\"Bottom\":[],\"Left\":[{\"id\":\"B\",\"label\":\"B\",\"type\":\"foundation.hydraulic.hydraulic\"}],\"Right\":[{\"id\":\"V\",\"label\":\"V\",\"type\":\"output\"},{\"id\":\"A\",\"label\":\"A\",\"type\":\"foundation.hydraulic.hydraulic\"}],\"Top\":[]}"
  Tank 2 (N13) : sh_lib/Low-Pressure Blocks/Tank  press=0 Pa  level_spec=1  tank_area=0.8 m^2  fluid_volume_tab=[0, .0028, .0065, .0114, .0176, .0252, .0344, .0436, .0512, .0574, .0623, .066, .0688, .0707, .072, .0727] m^3  fluid_level_tab=[0, .02, .04, .06, .08, .1, .12, .14, .16, .18, .2, .22, .24, .26, .28, .3] m  interp_method=1  extrap_method=1  pipe_diam=0.02 m  loss_coeff=1.2  g=9.80665 m/s^2  min_level=1e-3 m  fluid_level_check=0  volume_specify=off  volume_priority=High  volume=100 m^3  volume_nominal_specify=off  volume_nominal_unit=l  volume_nominal_value=1  level_specify=off  level_priority=None  level=station_2.fluid_level m  level_nominal_specify=off  level_nominal_unit=m  level_nominal_value=1  pipe_diam_A=0.20 m  loss_coeff_A=1.2  height_B=0.8 m  pipe_diam_B=0.23 m  loss_coeff_B=1.2  height_C=0.8 m  pipe_diam_C=0.02 m  loss_coeff_C=1.2
      settings: InternalSimscapePortConfiguration="{\"Bottom\":[],\"Left\":[{\"id\":\"B\",\"label\":\"B\",\"type\":\"foundation.hydraulic.hydraulic\"}],\"Right\":[{\"id\":\"V\",\"label\":\"V\",\"type\":\"output\"},{\"id\":\"A\",\"label\":\"A\",\"type\":\"foundation.hydraulic.hydraulic\"}],\"Top\":[]}"
  Tank1 : sh_lib/Low-Pressure Blocks/Tank  press=0 Pa  level_spec=1  tank_area=0.8 m^2  fluid_volume_tab=[0, .0028, .0065, .0114, .0176, .0252, .0344, .0436, .0512, .0574, .0623, .066, .0688, .0707, .072, .0727] m^3  fluid_level_tab=[0, .02, .04, .06, .08, .1, .12, .14, .16, .18, .2, .22, .24, .26, .28, .3] m  interp_method=1  extrap_method=1  pipe_diam=0.10 m  loss_coeff=1.2  g=9.80665 m/s^2  min_level=1e-3 m  fluid_level_check=0  volume_specify=off  volume_priority=High  volume=20 l  volume_nominal_specify=off  volume_nominal_unit=l  volume_nominal_value=1  level_specify=off  level_priority=None  level=0.025 m  level_nominal_specify=off  level_nominal_unit=m  level_nominal_value=1  pipe_diam_A=0.02 m  loss_coeff_A=1.2  height_B=0.8 m  pipe_diam_B=0.02 m  loss_coeff_B=1.2  height_C=0.8 m  pipe_diam_C=0.02 m  loss_coeff_C=1.2
      settings: InternalSimscapePortConfiguration="{\"Bottom\":[],\"Left\":[],\"Right\":[{\"id\":\"V\",\"label\":\"V\",\"type\":\"output\"},{\"id\":\"T\",\"label\":\"T\",\"type\":\"foundation.hydraulic.hydraulic\"}],\"Top\":[]}"
  Tank2 : sh_lib/Low-Pressure Blocks/Tank  press=0 Pa  level_spec=1  tank_area=0.8 m^2  fluid_volume_tab=[0, .0028, .0065, .0114, .0176, .0252, .0344, .0436, .0512, .0574, .0623, .066, .0688, .0707, .072, .0727] m^3  fluid_level_tab=[0, .02, .04, .06, .08, .1, .12, .14, .16, .18, .2, .22, .24, .26, .28, .3] m  interp_method=1  extrap_method=1  pipe_diam=0.10 m  loss_coeff=1.2  g=9.80665 m/s^2  min_level=1e-3 m  fluid_level_check=0  volume_specify=off  volume_priority=High  volume=20 l  volume_nominal_specify=off  volume_nominal_unit=l  volume_nominal_value=1  level_specify=off  level_priority=None  level=0.025 m  level_nominal_specify=off  level_nominal_unit=m  level_nominal_value=1  pipe_diam_A=0.02 m  loss_coeff_A=1.2  height_B=0.8 m  pipe_diam_B=0.02 m  loss_coeff_B=1.2  height_C=0.8 m  pipe_diam_C=0.02 m  loss_coeff_C=1.2
      settings: InternalSimscapePortConfiguration="{\"Bottom\":[],\"Left\":[],\"Right\":[{\"id\":\"V\",\"label\":\"V\",\"type\":\"output\"},{\"id\":\"T\",\"label\":\"T\",\"type\":\"foundation.hydraulic.hydraulic\"}],\"Top\":[]}"
  Three-Phase Parallel RLC Branch1 : spsThreePhaseParallelRLCBranchLib/Three-Phase Parallel RLC Branch  LConnTagsString=A|B|C  RConnTagsString=A|B|C  BranchType=R  Resistance=1000000  Inductance=1e-3  Capacitance=1e-6  Measurements=None
  Three-Phase Parallel RLC Branch2 : spsThreePhaseParallelRLCBranchLib/Three-Phase Parallel RLC Branch  LConnTagsString=A|B|C  RConnTagsString=A|B|C  BranchType=R  Resistance=1000000  Inductance=1e-3  Capacitance=1e-6  Measurements=None
  Three-Phase Parallel RLC Branch3 : spsThreePhaseParallelRLCBranchLib/Three-Phase Parallel RLC Branch  LConnTagsString=A|B|C  RConnTagsString=A|B|C  BranchType=R  Resistance=1000000  Inductance=1e-3  Capacitance=1e-6  Measurements=None
  Three-Phase Series RLC Branch : spsThreePhaseSeriesRLCBranchLib/Three-Phase Series RLC Branch  LConnTagsString=A|B|C  RConnTagsString=A|B|C  BranchType=RL  Resistance=0.0922  Inductance=0.0470/2/pi/50  Capacitance=1e-6  Measurements=None
  Three-Phase Series RLC Branch1 : spsThreePhaseSeriesRLCBranchLib/Three-Phase Series RLC Branch  LConnTagsString=A|B|C  RConnTagsString=A|B|C  BranchType=RL  Resistance=0.4930  Inductance=0.2511/2/pi/50  Capacitance=1e-6  Measurements=None
  Three-Phase Series RLC Branch10 : spsThreePhaseSeriesRLCBranchLib/Three-Phase Series RLC Branch  LConnTagsString=A|B|C  RConnTagsString=A|B|C  BranchType=RL  Resistance=0.3744  Inductance=0.1238/2/pi/50  Capacitance=1e-6  Measurements=None
  Three-Phase Series RLC Branch11 : spsThreePhaseSeriesRLCBranchLib/Three-Phase Series RLC Branch  LConnTagsString=A|B|C  RConnTagsString=A|B|C  BranchType=RL  Resistance=1.468  Inductance=1.155/2/pi/50  Capacitance=1e-6  Measurements=None
  Three-Phase Series RLC Branch12 : spsThreePhaseSeriesRLCBranchLib/Three-Phase Series RLC Branch  LConnTagsString=A|B|C  RConnTagsString=A|B|C  BranchType=RL  Resistance=0.5416  Inductance=0.7129/2/pi/50  Capacitance=1e-6  Measurements=None
  Three-Phase Series RLC Branch13 : spsThreePhaseSeriesRLCBranchLib/Three-Phase Series RLC Branch  LConnTagsString=A|B|C  RConnTagsString=A|B|C  BranchType=RL  Resistance=0.591  Inductance=0.526/2/pi/50  Capacitance=1e-6  Measurements=None
  Three-Phase Series RLC Branch14 : spsThreePhaseSeriesRLCBranchLib/Three-Phase Series RLC Branch  LConnTagsString=A|B|C  RConnTagsString=A|B|C  BranchType=RL  Resistance=0.7463  Inductance=0.545/2/pi/50  Capacitance=1e-6  Measurements=None
  Three-Phase Series RLC Branch15 : spsThreePhaseSeriesRLCBranchLib/Three-Phase Series RLC Branch  LConnTagsString=A|B|C  RConnTagsString=A|B|C  BranchType=RL  Resistance=1.289  Inductance=1.721/2/pi/50  Capacitance=1e-6  Measurements=None
  Three-Phase Series RLC Branch16 : spsThreePhaseSeriesRLCBranchLib/Three-Phase Series RLC Branch  LConnTagsString=A|B|C  RConnTagsString=A|B|C  BranchType=RL  Resistance=0.7320  Inductance=0.5740/2/pi/50  Capacitance=1e-6  Measurements=None
  Three-Phase Series RLC Branch17 : spsThreePhaseSeriesRLCBranchLib/Three-Phase Series RLC Branch  LConnTagsString=A|B|C  RConnTagsString=A|B|C  BranchType=RL  Resistance=0.164  Inductance=0.1565/2/pi/50  Capacitance=1e-6  Measurements=None
  Three-Phase Series RLC Branch18 : spsThreePhaseSeriesRLCBranchLib/Three-Phase Series RLC Branch  LConnTagsString=A|B|C  RConnTagsString=A|B|C  BranchType=RL  Resistance=1.5042  Inductance=1.3554/2/pi/50  Capacitance=1e-6  Measurements=None
  Three-Phase Series RLC Branch19 : spsThreePhaseSeriesRLCBranchLib/Three-Phase Series RLC Branch  LConnTagsString=A|B|C  RConnTagsString=A|B|C  BranchType=RL  Resistance=0.4095  Inductance=0.4784/2/pi/50  Capacitance=1e-6  Measurements=None
  Three-Phase Series RLC Branch2 : spsThreePhaseSeriesRLCBranchLib/Three-Phase Series RLC Branch  LConnTagsString=A|B|C  RConnTagsString=A|B|C  BranchType=RL  Resistance=0.366  Inductance=0.1864/2/pi/50  Capacitance=1e-6  Measurements=None
  Three-Phase Series RLC Branch20 : spsThreePhaseSeriesRLCBranchLib/Three-Phase Series RLC Branch  LConnTagsString=A|B|C  RConnTagsString=A|B|C  BranchType=RL  Resistance=0.7089  Inductance=0.9373/2/pi/50  Capacitance=1e-6  Measurements=None
  Three-Phase Series RLC Branch21 : spsThreePhaseSeriesRLCBranchLib/Three-Phase Series RLC Branch  LConnTagsString=A|B|C  RConnTagsString=A|B|C  BranchType=RL  Resistance=0.4512  Inductance=0.3083/2/pi/50  Capacitance=1e-6  Measurements=None
  Three-Phase Series RLC Branch22 : spsThreePhaseSeriesRLCBranchLib/Three-Phase Series RLC Branch  LConnTagsString=A|B|C  RConnTagsString=A|B|C  BranchType=RL  Resistance=0.8980  Inductance=0.7091/2/pi/50  Capacitance=1e-6  Measurements=None
  Three-Phase Series RLC Branch23 : spsThreePhaseSeriesRLCBranchLib/Three-Phase Series RLC Branch  LConnTagsString=A|B|C  RConnTagsString=A|B|C  BranchType=RL  Resistance=0.896  Inductance=0.7011/2/pi/50  Capacitance=1e-6  Measurements=None
  Three-Phase Series RLC Branch24 : spsThreePhaseSeriesRLCBranchLib/Three-Phase Series RLC Branch  LConnTagsString=A|B|C  RConnTagsString=A|B|C  BranchType=RL  Resistance=0.2030  Inductance=0.1034/2/pi/50  Capacitance=1e-6  Measurements=None
  Three-Phase Series RLC Branch25 : spsThreePhaseSeriesRLCBranchLib/Three-Phase Series RLC Branch  LConnTagsString=A|B|C  RConnTagsString=A|B|C  BranchType=RL  Resistance=0.2842  Inductance=0.1447/2/pi/50  Capacitance=1e-6  Measurements=None
  Three-Phase Series RLC Branch26 : spsThreePhaseSeriesRLCBranchLib/Three-Phase Series RLC Branch  LConnTagsString=A|B|C  RConnTagsString=A|B|C  BranchType=RL  Resistance=1.0590  Inductance=0.9337/2/pi/50  Capacitance=1e-6  Measurements=None
  Three-Phase Series RLC Branch27 : spsThreePhaseSeriesRLCBranchLib/Three-Phase Series RLC Branch  LConnTagsString=A|B|C  RConnTagsString=A|B|C  BranchType=RL  Resistance=0.8042  Inductance=0.7006/2/pi/50  Capacitance=1e-6  Measurements=None
  Three-Phase Series RLC Branch28 : spsThreePhaseSeriesRLCBranchLib/Three-Phase Series RLC Branch  LConnTagsString=A|B|C  RConnTagsString=A|B|C  BranchType=RL  Resistance=0.5075  Inductance=0.2585/2/pi/50  Capacitance=1e-6  Measurements=None
  Three-Phase Series RLC Branch29 : spsThreePhaseSeriesRLCBranchLib/Three-Phase Series RLC Branch  LConnTagsString=A|B|C  RConnTagsString=A|B|C  BranchType=RL  Resistance=0.9744  Inductance=0.963/2/pi/50  Capacitance=1e-6  Measurements=None
  Three-Phase Series RLC Branch3 : spsThreePhaseSeriesRLCBranchLib/Three-Phase Series RLC Branch  LConnTagsString=A|B|C  RConnTagsString=A|B|C  BranchType=RL  Resistance=0.3811  Inductance=0.1941/2/pi/50  Capacitance=1e-6  Measurements=None
  Three-Phase Series RLC Branch30 : spsThreePhaseSeriesRLCBranchLib/Three-Phase Series RLC Branch  LConnTagsString=A|B|C  RConnTagsString=A|B|C  BranchType=RL  Resistance=0.3105  Inductance=0.3619/2/pi/50  Capacitance=1e-6  Measurements=None
  Three-Phase Series RLC Branch31 : spsThreePhaseSeriesRLCBranchLib/Three-Phase Series RLC Branch  LConnTagsString=A|B|C  RConnTagsString=A|B|C  BranchType=RL  Resistance=0.341  Inductance=0.5302/2/pi/50  Capacitance=1e-6  Measurements=None
  Three-Phase Series RLC Branch4 : spsThreePhaseSeriesRLCBranchLib/Three-Phase Series RLC Branch  LConnTagsString=A|B|C  RConnTagsString=A|B|C  BranchType=RL  Resistance=0.819  Inductance=0.707/2/pi/50  Capacitance=1e-6  Measurements=None
  Three-Phase Series RLC Branch5 : spsThreePhaseSeriesRLCBranchLib/Three-Phase Series RLC Branch  LConnTagsString=A|B|C  RConnTagsString=A|B|C  BranchType=RL  Resistance=0.1872  Inductance=0.6188/2/pi/50  Capacitance=1e-6  Measurements=None
  Three-Phase Series RLC Branch6 : spsThreePhaseSeriesRLCBranchLib/Three-Phase Series RLC Branch  LConnTagsString=A|B|C  RConnTagsString=A|B|C  BranchType=RL  Resistance=0.7114  Inductance=0.2351/2/pi/50  Capacitance=1e-6  Measurements=None
  Three-Phase Series RLC Branch7 : spsThreePhaseSeriesRLCBranchLib/Three-Phase Series RLC Branch  LConnTagsString=A|B|C  RConnTagsString=A|B|C  BranchType=RL  Resistance=1.0300  Inductance=0.74/2/pi/50  Capacitance=1e-6  Measurements=None
  Three-Phase Series RLC Branch8 : spsThreePhaseSeriesRLCBranchLib/Three-Phase Series RLC Branch  LConnTagsString=A|B|C  RConnTagsString=A|B|C  BranchType=RL  Resistance=1.044  Inductance=0.74/2/pi/50  Capacitance=1e-6  Measurements=None
  Three-Phase Series RLC Branch9 : spsThreePhaseSeriesRLCBranchLib/Three-Phase Series RLC Branch  LConnTagsString=A|B|C  RConnTagsString=A|B|C  BranchType=RL  Resistance=1.044  Inductance=0.74/2/pi/50  Capacitance=1e-6  Measurements=None
  Three-Phase V-I Measurement1 : spsThreePhaseVIMeasurementLib/Three-Phase V-I Measurement  VoltageMeasurement=phase-to-ground  SetLabelV=off  LabelV=Vabc  Vpu=off  VpuLL=off  CurrentMeasurement=yes  SetLabelI=off  LabelI=Iabc  Ipu=off  Pbase=100e6  Vbase=500e3  OutputType=Complex  PhasorSimulation=off  PSBequivalent=0
  Three-Phase V-I Measurement2 : spsThreePhaseVIMeasurementLib/Three-Phase V-I Measurement  VoltageMeasurement=phase-to-ground  SetLabelV=off  LabelV=Vabc  Vpu=off  VpuLL=off  CurrentMeasurement=yes  SetLabelI=off  LabelI=Iabc  Ipu=off  Pbase=100e6  Vbase=500e3  OutputType=Complex  PhasorSimulation=off  PSBequivalent=0
  Three-Phase V-I Measurement3 : spsThreePhaseVIMeasurementLib/Three-Phase V-I Measurement  VoltageMeasurement=phase-to-ground  SetLabelV=off  LabelV=Vabc  Vpu=off  VpuLL=off  CurrentMeasurement=yes  SetLabelI=off  LabelI=Iabc  Ipu=off  Pbase=100e6  Vbase=500e3  OutputType=Complex  PhasorSimulation=off  PSBequivalent=0
  Three-Phase Fault : spsThreePhaseFaultLib/Three-Phase Fault  InitialStates=0  FaultA=on  FaultB=on  FaultC=on  GroundFault=on  SwitchTimes="[900  1500]"  External=off  SwitchStatus=NaN  FaultResistance=-0.002  GroundResistance=1e-6  SnubberResistance=1e6  SnubberCapacitance=inf  Measurements=None
  Three-Phase Fault1 : spsThreePhaseFaultLib/Three-Phase Fault  InitialStates=0  FaultA=on  FaultB=on  FaultC=on  GroundFault=on  SwitchTimes="[900  1500]"  External=off  SwitchStatus=NaN  FaultResistance=-0.002  GroundResistance=1e-6  SnubberResistance=1e6  SnubberCapacitance=inf  Measurements=None
  Three-Phase Fault2 : spsThreePhaseFaultLib/Three-Phase Fault  InitialStates=0  FaultA=on  FaultB=on  FaultC=on  GroundFault=on  SwitchTimes="[900  1500]"  External=off  SwitchStatus=NaN  FaultResistance=-0.002  GroundResistance=1e-6  SnubberResistance=1e6  SnubberCapacitance=inf  Measurements=None
  Three-Phase Source : spsThreePhaseSourceLib/Three-Phase Source  InternalConnection=Yg  VoltagePhases=off  Voltage=12660  PhaseAngle=0  Voltage_phases=[25e3 25e3 25e3]/sqrt(3)  PhaseAngles_phases=[0 -120 +120]  Frequency=50  NonIdealSource=on  SpecifyImpedance=on  Resistance=0.8929  Inductance=16.58e-3  ShortCircuitLevel=100e6  BaseVoltage=12660  XRratio=7  BusType=swing  Pref=10e3  Qref=0  Prefabc=[10e3, 10e3, 10e3]  Qrefabc=[0, 0, 0]  Qmin=-inf  Qmax=inf
  Universal Bridge : spsUniversalBridgeLib/Universal Bridge  Arms=3  SnubberResistance=1e5  SnubberCapacitance=inf  Device=Diodes  Ron=1e-3  Lon=0  ForwardVoltages="[  0  0  ]"  ForwardVoltage=0  GTOparameters=[ 10e-6 , 20e-6 ]  IGBTparameters=[ 1e-6 , 2e-6 ]  Measurements=None  Measurements_2=None  converterType=Rectifier
  Universal Bridge1 : spsUniversalBridgeLib/Universal Bridge  Arms=3  SnubberResistance=1e5  SnubberCapacitance=inf  Device=Diodes  Ron=1e-3  Lon=0  ForwardVoltages="[  0  0  ]"  ForwardVoltage=0  GTOparameters=[ 10e-6 , 20e-6 ]  IGBTparameters=[ 1e-6 , 2e-6 ]  Measurements=None  Measurements_2=None  converterType=Rectifier
  Universal Bridge2 : spsUniversalBridgeLib/Universal Bridge  Arms=3  SnubberResistance=1e5  SnubberCapacitance=inf  Device=Diodes  Ron=1e-3  Lon=0  ForwardVoltages="[  0  0  ]"  ForwardVoltage=0  GTOparameters=[ 10e-6 , 20e-6 ]  IGBTparameters=[ 1e-6 , 2e-6 ]  Measurements=None  Measurements_2=None  converterType=Rectifier
  "Voltage (3Φ, Re-Im)" : Scope
  "Voltage (3Φ, Re-Im)1" : Scope
  "Voltage (3Φ, Re-Im)2" : Scope
  Voltage Sensor : fl_lib/Electrical/Electrical Sensors/Voltage Sensor
  Voltage Sensor1 : fl_lib/Electrical/Electrical Sensors/Voltage Sensor
  Voltage Sensor2 : fl_lib/Electrical/Electrical Sensors/Voltage Sensor
  Volume (m^3) : Display
  Volume T1 : Subsystem
  Volume T2 : Subsystem
  Volume T3 : Subsystem
  Volume T4 : Subsystem
  Volume T5 : Subsystem
  Volume T6 : Subsystem
  Water Properties : sh_lib/Hydraulic Utilities/Hydraulic Fluid  SelFluid=24  SysTemp=1  TrapAir=0.001  ViscDerFactor=1  range_error=2
  powergui : spspowerguiLib/powergui  Priority=1  SimulationMode=Discrete  SampleTime=0.25  frequency=50  Iterations=50  frequencyindice=0  Pbase=100e6  ErrMax=1e-4  UnitsV=kV  UnitsW=MW  buscounter=0  FunctionMessages=off  echomessages=off  EnableUseOfTLC=off  CurrentSourceSwitches=off  DisableSnubberDevices=off  DisableRonSwitches=off  DisableVfSwitches=off  DisplayEquations=off  AutomaticDiscreteSolvers=off  SolverType=Tustin/Backward Euler (TBE)  Interpol=off  ExternalGateDelay=off  methode=off  Ts=100  x0status=blocks  SPID=on  SwTol=0  HookPort=off  NonlinearTolerance=1e-4  nMaxIteration=100  ContinueOnMaxIteration=off  RestoreLinks=warning  ResistiveCurrentMeasurement=off  Frange=[0:2:500]  Ylog=off  Xlog=on  ShowGrid=off  save=off  variable=ZData  structure=0  ZoomFFT=off  StartTime=0.0  cycles=1  DisplayStyle=1  fundamental=60  FreqAxis=off  MaxFrequency=1000  frequencyindicesteady=1  RmsSteady=1  display=off
  tag scope: W_PSS1=global, W_PSS2=global, W_PSS3=global
  wires:
  [V_S4] -> Mux1/3
  [V_S5] -> Mux2/2
  [V_S3] -> Mux1/2
  [V_S2] -> Mux/2
  [V_S6] -> Mux1/5
  [V_S5] -> Mux1/4
  [V_S1] -> Mux/1
  Mux/1 -> Scope/1
  [V_S4] -> Mux2/1
  [V_S3] -> Mux/3
  Mux1/1 -> Volume (m^3)/1
  [V_S2] -> Mux1/1
  [V_S6] -> Mux2/3
  Constant1/1 -> Product1/2
  "Power (3ph, Phasor)1"/1 -> Real Power1/1
  Product1/1 -> Saturation2/1
  Product2/1 -> Saturation1/1
  "Power (3ph, Phasor)2"/1 -> Real Power2/1
  PS-Simulink Converter4/1 -> DC voltage2/1, Display2/1
  Product/1 -> Saturation/1
  Three-Phase V-I Measurement3/1 -> "Voltage (3Φ, Re-Im)2"/1, "Power (3ph, Phasor)2"/1
  Constant2/1 -> Product2/2
  PS-Simulink Converter2/1 -> DC voltage1/1, Display1/1
  PS-Simulink Converter1/1 -> Product/1
  Three-Phase V-I Measurement1/2 -> "Power (3ph, Phasor)"/2
  PS-Simulink Converter5/1 -> Product2/1
  Three-Phase V-I Measurement3/2 -> "Power (3ph, Phasor)2"/2
  Three-Phase V-I Measurement1/1 -> "Voltage (3Φ, Re-Im)"/1, "Power (3ph, Phasor)"/1
  Three-Phase V-I Measurement2/2 -> "Power (3ph, Phasor)1"/2
  PS-Simulink Converter/1 -> DC voltage/1, Display/1
  Three-Phase V-I Measurement2/1 -> "Voltage (3Φ, Re-Im)1"/1, "Power (3ph, Phasor)1"/1
  "Power (3ph, Phasor)"/1 -> Real Power/1
  PS-Simulink Converter3/1 -> Product1/1
  Constant/1 -> Product/2
  Saturation/1 -> Scope1/1, [W_PSS2], RPM/1
  Saturation1/1 -> Scope3/1, [W_PSS3], RPM2/1
  Saturation2/1 -> Scope2/1, [W_PSS1], RPM1/1
  Mux2/1 -> Scope/2
  connections:
  Hydraulic Pipeline/LConn1 -- Subsystem/LConn1 -- Hydraulic Pipeline1/RConn1
  Hydraulic Pipeline5/LConn1 -- Hydraulic Pipeline4/RConn1 -- Hydraulic Pipeline9/LConn1
  Water Properties/RConn1 -- Reservoir (Node 1)/LConn2 -- Reservoir (Node 1)/LConn3 -- Pump Station 1/LConn1 -- Solver Configuration1/RConn1
  Hydraulic Pipeline11/LConn1 -- Hydraulic Pipeline10/RConn1
  Hydraulic Pipeline8/LConn1 -- Tank 1 (N10)/LConn1
  Tank1/RConn2 -- Subsystem/RConn1
  Pump Station 1/RConn1 -- Hydraulic Pipeline2/LConn1
  Hydraulic Pipeline2/RConn1 -- Hydraulic Pipeline1/LConn1
  Pump Station 2/RConn1 -- Hydraulic Pipeline3/LConn1
  Hydraulic Pipeline8/RConn1 -- Subsystem2/LConn1
  Volume T1/LConn1 -- Reservoir (Node 1)/LConn1
  Tank1/RConn1 -- Volume T4/LConn1
  Hydraulic Pipeline/RConn1 -- Pump Station 2/LConn1
  Hydraulic Pipeline7/RConn1 -- Tank 1 (N10)/RConn2
  Hydraulic Pipeline10/LConn1 -- Tank 2 (N13)/LConn1
  Hydraulic Pipeline4/LConn1 -- Hydraulic Pipeline3/RConn1
  Hydraulic Pipeline7/LConn1 -- Hydraulic Pipeline6/RConn1
  Volume T3/LConn1 -- Tank 2 (N13)/RConn1
  Subsystem1/RConn1 -- Tank/RConn2
  Tank2/RConn1 -- Volume T5/LConn1
  Tank/RConn1 -- Volume T6/LConn1
  Pump Station 3/RConn1 -- Hydraulic Pipeline6/LConn1
  Pump Station 3/LConn1 -- Hydraulic Pipeline5/RConn1
  Tank2/RConn2 -- Subsystem2/RConn1
  Hydraulic Pipeline9/RConn1 -- Tank 2 (N13)/RConn2
  Hydraulic Pipeline11/RConn1 -- Subsystem1/LConn1
  Volume T2/LConn1 -- Tank 1 (N10)/RConn1
  Generic Rotary Actuator/LConn2 -- Rotational Damper/RConn1 -- Ideal Rotational Motion Sensor/LConn1
  Three-Phase V-I Measurement1/LConn3 -- Bus_22/RConn3 -- Three-Phase Fault/LConn3 -- Three-Phase Parallel RLC Branch1/LConn3
  Ideal Rotational Motion Sensor1/LConn1 -- Generic Rotary Actuator1/LConn2 -- Rotational Damper1/RConn1
  Generic Rotary Actuator/LConn1 -- Voltage Sensor/LConn1 -- Solver Configuration3/RConn1 -- Current-Voltage Simscape Interface (gnd)1/RConn1
  Three-Phase Parallel RLC Branch3/RConn2 -- Three-Phase Parallel RLC Branch3/RConn1 -- Ground2/LConn1 -- Three-Phase Parallel RLC Branch3/RConn3
  Bus_33/RConn3 -- Three-Phase Fault2/LConn3 -- Three-Phase V-I Measurement3/LConn3 -- Three-Phase Parallel RLC Branch3/LConn3
  Three-Phase V-I Measurement2/LConn2 -- Bus_18/RConn2 -- Three-Phase Fault1/LConn2 -- Three-Phase Parallel RLC Branch2/LConn2
  Three-Phase V-I Measurement2/LConn3 -- Three-Phase Fault1/LConn3 -- Bus_18/RConn3 -- Three-Phase Parallel RLC Branch2/LConn3
  Three-Phase Parallel RLC Branch2/LConn1 -- Three-Phase V-I Measurement2/LConn1 -- Bus_18/RConn1 -- Three-Phase Fault1/LConn1
  Three-Phase V-I Measurement1/LConn2 -- Bus_22/RConn2 -- Three-Phase Fault/LConn2 -- Three-Phase Parallel RLC Branch1/LConn2
  Solver Configuration2/RConn1 -- Current-Voltage Simscape Interface (gnd)3/RConn1 -- Voltage Sensor1/LConn1 -- Generic Rotary Actuator1/LConn1
  Three-Phase Parallel RLC Branch1/LConn1 -- Three-Phase V-I Measurement1/LConn1 -- Bus_22/RConn1 -- Three-Phase Fault/LConn1
  Generic Rotary Actuator/RConn2 -- Mechanical Rotational Reference/LConn1 -- Ideal Rotational Motion Sensor/RConn1
  Ideal Rotational Motion Sensor2/LConn1 -- Generic Rotary Actuator2/LConn2 -- Rotational Damper2/RConn1
  Generic Rotary Actuator2/LConn1 -- Current-Voltage Simscape Interface (gnd)5/RConn1 -- Solver Configuration4/RConn1 -- Voltage Sensor2/LConn1
  Three-Phase Parallel RLC Branch3/LConn1 -- Bus_33/RConn1 -- Three-Phase Fault2/LConn1 -- Three-Phase V-I Measurement3/LConn1
  Bus_33/RConn2 -- Three-Phase Fault2/LConn2 -- Three-Phase V-I Measurement3/LConn2 -- Three-Phase Parallel RLC Branch3/LConn2
  Ideal Rotational Motion Sensor1/RConn1 -- Generic Rotary Actuator1/RConn2 -- Mechanical Rotational Reference1/LConn1
  Ideal Rotational Motion Sensor2/RConn1 -- Generic Rotary Actuator2/RConn2 -- Mechanical Rotational Reference2/LConn1
  Current-Voltage Simscape Interface (gnd)6/RConn1 -- Generic Rotary Actuator2/RConn1 -- Voltage Sensor2/RConn2
  Current-Voltage Simscape Interface (gnd)4/RConn1 -- Generic Rotary Actuator1/RConn1 -- Voltage Sensor1/RConn2
  Three-Phase Parallel RLC Branch2/RConn2 -- Three-Phase Parallel RLC Branch2/RConn1 -- Ground1/LConn1 -- Three-Phase Parallel RLC Branch2/RConn3
  Three-Phase Parallel RLC Branch1/RConn2 -- Three-Phase Parallel RLC Branch1/RConn3 -- Ground/LConn1 -- Three-Phase Parallel RLC Branch1/RConn1
  Generic Rotary Actuator/RConn1 -- Voltage Sensor/RConn2 -- Current-Voltage Simscape Interface (gnd)2/RConn1
  Three-Phase Source/RConn1 -- Bus_1/LConn1
  Bus_33/LConn2 -- Three-Phase Series RLC Branch31/RConn2
  Three-Phase Series RLC Branch/RConn3 -- Bus_2/LConn3
  Bus_24/LConn1 -- Three-Phase Series RLC Branch22/RConn1
  Bus_23/LConn1 -- Three-Phase Series RLC Branch21/RConn1
  Bus_7/LConn2 -- Three-Phase Series RLC Branch5/RConn2
  Bus_31/LConn2 -- Three-Phase Series RLC Branch29/RConn2
  PS-Simulink Converter3/LConn1 -- Ideal Rotational Motion Sensor1/RConn2
  Bus_16/LConn2 -- Three-Phase Series RLC Branch14/RConn2
  Three-Phase Series RLC Branch13/LConn3 -- Bus_14/RConn3
  Bus_23/LConn3 -- Three-Phase Series RLC Branch21/RConn3
  Bus_30/RConn2 -- Three-Phase Series RLC Branch29/LConn1
  Bus_31/RConn3 -- Three-Phase Series RLC Branch30/LConn3
  Three-Phase Series RLC Branch6/LConn3 -- Bus_7/RConn3
  Three-Phase V-I Measurement2/RConn2 -- Universal Bridge1/LConn2
  Three-Phase Series RLC Branch8/LConn3 -- Bus_9/RConn3
  Three-Phase Series RLC Branch/RConn1 -- Bus_2/LConn1
  Bus_26/LConn1 -- Three-Phase Series RLC Branch24/RConn1
  Bus_27/RConn1 -- Three-Phase Series RLC Branch26/LConn1
  Bus_19/LConn1 -- Three-Phase Series RLC Branch17/RConn1
  Bus_29/LConn1 -- Three-Phase Series RLC Branch27/RConn1
  Three-Phase Series RLC Branch4/RConn2 -- Bus_6/LConn2
  Bus_31/LConn1 -- Three-Phase Series RLC Branch29/RConn1
  Bus_21/LConn1 -- Three-Phase Series RLC Branch19/RConn1
  Three-Phase Series RLC Branch9/LConn2 -- Bus_10/RConn2
  Bus_30/RConn1 -- Three-Phase Series RLC Branch29/LConn2
  Three-Phase Series RLC Branch18/LConn2 -- Bus_19/RConn2
  Three-Phase Series RLC Branch14/LConn2 -- Bus_15/RConn2
  Universal Bridge1/RConn2 -- Current-Voltage Simscape Interface (gnd)4/LConn1
  Three-Phase Series RLC Branch5/LConn3 -- Bus_6/RConn6
  Bus_8/LConn3 -- Three-Phase Series RLC Branch6/RConn3
  Bus_12/LConn2 -- Three-Phase Series RLC Branch10/RConn2
  Bus_20/LConn3 -- Three-Phase Series RLC Branch18/RConn3
  Three-Phase Series RLC Branch19/LConn1 -- Bus_20/RConn1
  Bus_27/LConn2 -- Three-Phase Series RLC Branch25/RConn2
  Bus_10/LConn1 -- Three-Phase Series RLC Branch8/RConn1
  Bus_31/LConn3 -- Three-Phase Series RLC Branch29/RConn3
  Three-Phase Series RLC Branch7/RConn2 -- Bus_9/LConn2
  Bus_15/LConn1 -- Three-Phase Series RLC Branch13/RConn1
  Three-Phase Series RLC Branch1/LConn2 -- Bus_2/RConn2
  Three-Phase Series RLC Branch7/RConn1 -- Bus_9/LConn1
  Three-Phase Series RLC Branch7/LConn1 -- Bus_8/RConn1
  Bus_6/RConn1 -- Three-Phase Series RLC Branch24/LConn1
  Bus_19/LConn3 -- Three-Phase Series RLC Branch17/RConn3
  Bus_13/LConn3 -- Three-Phase Series RLC Branch11/RConn3
  Universal Bridge/RConn1 -- Current-Voltage Simscape Interface (gnd)1/LConn1
  Bus_14/LConn2 -- Three-Phase Series RLC Branch12/RConn2
  Three-Phase Series RLC Branch10/LConn3 -- Bus_11/RConn3
  Three-Phase Series RLC Branch5/LConn2 -- Bus_6/RConn5
  Three-Phase Series RLC Branch4/LConn3 -- Bus_5/RConn3
  Bus_29/LConn3 -- Three-Phase Series RLC Branch27/RConn3
  PS-Simulink Converter1/LConn1 -- Ideal Rotational Motion Sensor/RConn2
  Bus_31/RConn2 -- Three-Phase Series RLC Branch30/LConn2
  Three-Phase Series RLC Branch2/LConn1 -- Bus_3/RConn4
  Three-Phase Series RLC Branch16/LConn3 -- Bus_17/RConn3
  Bus_19/LConn2 -- Three-Phase Series RLC Branch17/RConn2
  Bus_23/RConn1 -- Three-Phase Series RLC Branch22/LConn2
  Three-Phase Series RLC Branch11/LConn3 -- Bus_12/RConn3
  Three-Phase Series RLC Branch8/LConn2 -- Bus_9/RConn2
  Bus_6/RConn3 -- Three-Phase Series RLC Branch24/LConn3
  Universal Bridge1/LConn1 -- Three-Phase V-I Measurement2/RConn1
  Bus_24/LConn3 -- Three-Phase Series RLC Branch22/RConn3
  Bus_29/RConn2 -- Three-Phase Series RLC Branch28/LConn2
  Bus_15/LConn2 -- Three-Phase Series RLC Branch13/RConn2
  Bus_4/LConn2 -- Three-Phase Series RLC Branch2/RConn2
  Bus_32/LConn1 -- Three-Phase Series RLC Branch30/RConn1
  Bus_32/LConn2 -- Three-Phase Series RLC Branch30/RConn2
  Three-Phase Series RLC Branch20/LConn1 -- Bus_21/RConn1
  Universal Bridge2/RConn1 -- Current-Voltage Simscape Interface (gnd)5/LConn1
  Three-Phase Series RLC Branch11/LConn2 -- Bus_12/RConn2
  Bus_13/LConn2 -- Three-Phase Series RLC Branch11/RConn2
  Bus_26/LConn2 -- Three-Phase Series RLC Branch24/RConn2
  Bus_17/LConn3 -- Three-Phase Series RLC Branch15/RConn3
  Bus_8/LConn1 -- Three-Phase Series RLC Branch6/RConn1
  Three-Phase Series RLC Branch12/LConn2 -- Bus_13/RConn2
  Three-Phase Series RLC Branch4/LConn1 -- Bus_5/RConn1
  Three-Phase Series RLC Branch15/LConn3 -- Bus_16/RConn3
  Universal Bridge/RConn2 -- Current-Voltage Simscape Interface (gnd)2/LConn1
  Three-Phase Series RLC Branch2/LConn3 -- Bus_3/RConn6
  Three-Phase Series RLC Branch10/LConn2 -- Bus_11/RConn2
  Bus_16/LConn3 -- Three-Phase Series RLC Branch14/RConn3
  Three-Phase Series RLC Branch2/LConn2 -- Bus_3/RConn5
  Bus_17/LConn2 -- Three-Phase Series RLC Branch15/RConn2
  Bus_25/LConn1 -- Three-Phase Series RLC Branch23/RConn1
  Three-Phase Series RLC Branch19/LConn2 -- Bus_20/RConn2
  Rotational Damper2/LConn1 -- Inertia2/LConn1
  Bus_26/RConn3 -- Three-Phase Series RLC Branch25/LConn3
  Three-Phase Series RLC Branch13/LConn1 -- Bus_14/RConn1
  Bus_3/LConn3 -- Three-Phase Series RLC Branch1/RConn3
  Three-Phase Series RLC Branch14/LConn3 -- Bus_15/RConn3
  Bus_27/RConn3 -- Three-Phase Series RLC Branch26/LConn3
  Three-Phase V-I Measurement1/RConn2 -- Universal Bridge/LConn2
  Bus_22/LConn1 -- Three-Phase Series RLC Branch20/RConn1
  Bus_1/RConn1 -- Three-Phase Series RLC Branch/LConn1
  Three-Phase Series RLC Branch9/LConn3 -- Bus_10/RConn3
  Three-Phase Series RLC Branch5/LConn1 -- Bus_6/RConn4
  Three-Phase Series RLC Branch3/LConn1 -- Bus_4/RConn1
  Bus_27/LConn3 -- Three-Phase Series RLC Branch25/RConn3
  Three-Phase Series RLC Branch15/LConn1 -- Bus_16/RConn1
  Universal Bridge2/RConn2 -- Current-Voltage Simscape Interface (gnd)6/LConn1
  Bus_26/LConn3 -- Three-Phase Series RLC Branch24/RConn3
  Bus_17/LConn1 -- Three-Phase Series RLC Branch15/RConn1
  Bus_14/LConn1 -- Three-Phase Series RLC Branch12/RConn1
  Bus_2/RConn5 -- Three-Phase Series RLC Branch17/LConn2
  Bus_4/LConn1 -- Three-Phase Series RLC Branch2/RConn1
  Universal Bridge2/LConn1 -- Three-Phase V-I Measurement3/RConn1
  Three-Phase Series RLC Branch6/LConn1 -- Bus_7/RConn1
  Three-Phase Series RLC Branch1/RConn1 -- Bus_3/LConn1
  Three-Phase Series RLC Branch12/LConn3 -- Bus_13/RConn3
  Bus_11/LConn2 -- Three-Phase Series RLC Branch9/RConn2
  Bus_2/RConn4 -- Three-Phase Series RLC Branch17/LConn1
  Bus_15/LConn3 -- Three-Phase Series RLC Branch13/RConn3
  Three-Phase Series RLC Branch18/LConn3 -- Bus_19/RConn3
  Bus_6/LConn3 -- Three-Phase Series RLC Branch4/RConn3
  Bus_26/RConn1 -- Three-Phase Series RLC Branch25/LConn1
  Bus_20/LConn1 -- Three-Phase Series RLC Branch18/RConn1
  Bus_4/LConn3 -- Three-Phase Series RLC Branch2/RConn3
  Bus_10/LConn2 -- Three-Phase Series RLC Branch8/RConn2
  Bus_30/LConn2 -- Three-Phase Series RLC Branch28/RConn2
  Three-Phase Series RLC Branch7/LConn3 -- Bus_8/RConn3
  Three-Phase Series RLC Branch4/LConn2 -- Bus_5/RConn2
  Bus_26/RConn2 -- Three-Phase Series RLC Branch25/LConn2
  Three-Phase Series RLC Branch1/RConn2 -- Bus_3/LConn2
  Bus_21/LConn3 -- Three-Phase Series RLC Branch19/RConn3
  Three-Phase Series RLC Branch15/LConn2 -- Bus_16/RConn2
  Bus_32/LConn3 -- Three-Phase Series RLC Branch30/RConn3
  Three-Phase Series RLC Branch11/LConn1 -- Bus_12/RConn1
  Three-Phase Series RLC Branch10/LConn1 -- Bus_11/RConn1
  Bus_16/LConn1 -- Three-Phase Series RLC Branch14/RConn1
  Bus_6/RConn2 -- Three-Phase Series RLC Branch24/LConn2
  Three-Phase Series RLC Branch3/LConn3 -- Bus_4/RConn3
  Bus_24/RConn3 -- Three-Phase Series RLC Branch23/LConn3
  PS-Simulink Converter4/LConn1 -- Voltage Sensor2/RConn1
  Bus_23/RConn2 -- Three-Phase Series RLC Branch22/LConn1
  Bus_5/LConn3 -- Three-Phase Series RLC Branch3/RConn3
  Bus_12/LConn3 -- Three-Phase Series RLC Branch10/RConn3
  Bus_30/LConn1 -- Three-Phase Series RLC Branch28/RConn1
  Three-Phase Source/RConn3 -- Bus_1/LConn3
  Bus_30/LConn3 -- Three-Phase Series RLC Branch28/RConn3
  Three-Phase Series RLC Branch6/LConn2 -- Bus_7/RConn2
  Three-Phase Series RLC Branch21/LConn3 -- Bus_3/RConn3
  Bus_25/LConn2 -- Three-Phase Series RLC Branch23/RConn2
  Bus_32/RConn3 -- Three-Phase Series RLC Branch31/LConn3
  Three-Phase V-I Measurement3/RConn3 -- Universal Bridge2/LConn3
  Bus_5/LConn1 -- Three-Phase Series RLC Branch3/RConn1
  Bus_22/LConn2 -- Three-Phase Series RLC Branch20/RConn2
  Bus_10/LConn3 -- Three-Phase Series RLC Branch8/RConn3
  Three-Phase Series RLC Branch/RConn2 -- Bus_2/LConn2
  Bus_1/RConn3 -- Three-Phase Series RLC Branch/LConn3
  Bus_24/LConn2 -- Three-Phase Series RLC Branch22/RConn2
  Three-Phase Series RLC Branch18/LConn1 -- Bus_19/RConn1
  Three-Phase Series RLC Branch21/LConn1 -- Bus_3/RConn1
  Universal Bridge/LConn1 -- Three-Phase V-I Measurement1/RConn1
  Three-Phase Series RLC Branch13/LConn2 -- Bus_14/RConn2
  Bus_11/LConn1 -- Three-Phase Series RLC Branch9/RConn1
  PS-Simulink Converter/LConn1 -- Voltage Sensor/RConn1
  Three-Phase Series RLC Branch12/LConn1 -- Bus_13/RConn1
  Three-Phase Series RLC Branch7/LConn2 -- Bus_8/RConn2
  Bus_27/LConn1 -- Three-Phase Series RLC Branch25/RConn1
  Three-Phase V-I Measurement3/RConn2 -- Universal Bridge2/LConn2
  Three-Phase Series RLC Branch20/LConn3 -- Bus_21/RConn3
  Bus_32/RConn2 -- Three-Phase Series RLC Branch31/LConn2
  Three-Phase Series RLC Branch16/LConn1 -- Bus_17/RConn1
  Bus_5/LConn2 -- Three-Phase Series RLC Branch3/RConn2
  Bus_18/LConn3 -- Three-Phase Series RLC Branch16/RConn3
  Bus_7/LConn1 -- Three-Phase Series RLC Branch5/RConn1
  Rotational Damper/LConn1 -- Inertia/LConn1
  Bus_7/LConn3 -- Three-Phase Series RLC Branch5/RConn3
  Bus_28/LConn3 -- Three-Phase Series RLC Branch26/RConn3
  Bus_8/LConn2 -- Three-Phase Series RLC Branch6/RConn2
  Bus_1/RConn2 -- Three-Phase Series RLC Branch/LConn2
  Three-Phase Series RLC Branch7/RConn3 -- Bus_9/LConn3
  Three-Phase Series RLC Branch21/LConn2 -- Bus_3/RConn2
  Bus_31/RConn1 -- Three-Phase Series RLC Branch30/LConn1
  Bus_2/RConn6 -- Three-Phase Series RLC Branch17/LConn3
  Bus_28/RConn2 -- Three-Phase Series RLC Branch27/LConn2
  Three-Phase Series RLC Branch14/LConn1 -- Bus_15/RConn1
  Bus_28/LConn2 -- Three-Phase Series RLC Branch26/RConn2
  Three-Phase Series RLC Branch16/LConn2 -- Bus_17/RConn2
  Universal Bridge1/RConn1 -- Current-Voltage Simscape Interface (gnd)3/LConn1
  Bus_20/LConn2 -- Three-Phase Series RLC Branch18/RConn2
  Three-Phase V-I Measurement2/RConn3 -- Universal Bridge1/LConn3
  Bus_18/LConn2 -- Three-Phase Series RLC Branch16/RConn2
  Bus_24/RConn1 -- Three-Phase Series RLC Branch23/LConn1
  Three-Phase V-I Measurement1/RConn3 -- Universal Bridge/LConn3
  Bus_29/LConn2 -- Three-Phase Series RLC Branch27/RConn2
  Bus_28/RConn1 -- Three-Phase Series RLC Branch27/LConn1
  Bus_28/LConn1 -- Three-Phase Series RLC Branch26/RConn1
  Bus_22/LConn3 -- Three-Phase Series RLC Branch20/RConn3
  Bus_23/LConn2 -- Three-Phase Series RLC Branch21/RConn2
  Bus_33/LConn1 -- Three-Phase Series RLC Branch31/RConn1
  PS-Simulink Converter2/LConn1 -- Voltage Sensor1/RConn1
  Three-Phase Series RLC Branch1/LConn3 -- Bus_2/RConn3
  Bus_33/LConn3 -- Three-Phase Series RLC Branch31/RConn3
  Bus_23/RConn3 -- Three-Phase Series RLC Branch22/LConn3
  Three-Phase Series RLC Branch8/LConn1 -- Bus_9/RConn1
  Three-Phase Series RLC Branch19/LConn3 -- Bus_20/RConn3
  Bus_13/LConn1 -- Three-Phase Series RLC Branch11/RConn1
  Bus_30/RConn3 -- Three-Phase Series RLC Branch29/LConn3
  PS-Simulink Converter5/LConn1 -- Ideal Rotational Motion Sensor2/RConn2
  Bus_25/LConn3 -- Three-Phase Series RLC Branch23/RConn3
  Bus_21/LConn2 -- Three-Phase Series RLC Branch19/RConn2
  Bus_11/LConn3 -- Three-Phase Series RLC Branch9/RConn3
  Three-Phase Series RLC Branch4/RConn1 -- Bus_6/LConn1
  Bus_32/RConn1 -- Three-Phase Series RLC Branch31/LConn1
  Bus_18/LConn1 -- Three-Phase Series RLC Branch16/RConn1
  Bus_14/LConn3 -- Three-Phase Series RLC Branch12/RConn3
  Bus_12/LConn1 -- Three-Phase Series RLC Branch10/RConn1
  Three-Phase Series RLC Branch9/LConn1 -- Bus_10/RConn1
  Three-Phase Series RLC Branch3/LConn2 -- Bus_4/RConn2
  Bus_27/RConn2 -- Three-Phase Series RLC Branch26/LConn2
  Bus_28/RConn3 -- Three-Phase Series RLC Branch27/LConn3
  Three-Phase Source/RConn2 -- Bus_1/LConn2
  Three-Phase Series RLC Branch1/LConn1 -- Bus_2/RConn1
  Bus_24/RConn2 -- Three-Phase Series RLC Branch23/LConn2
  Bus_29/RConn3 -- Three-Phase Series RLC Branch28/LConn3
  Bus_29/RConn1 -- Three-Phase Series RLC Branch28/LConn1
  Three-Phase Series RLC Branch20/LConn2 -- Bus_21/RConn2
